simulink model "Wanderwellen_Leitungsmodell"  (R2022a)
settings: Solver=VariableStepAuto  StartTime=0.0  StopTime=0.05  RelTol=1e-3
model workspace (MAT data in the model file):
  C_impedanz = 1
  C_quelle = 1
  Delta_C = 2e-09
  Delta_G = 5000000
  Delta_L = 0.000228
  Delta_R = 0.048
  L_impedanz = 1
  L_quelle = 1
  R_impedanz = 0
  R_quelle = 0
  U = 20000
  U_type = 1
  Z_abschluss_type = 1
  Z_quelle_type = 1
  f = 50
  laenge = 0.2
  n_seg = 1
libraries: fl_lib x617, nesl_utility x207, ee_lib x3
(part 1 of 6)
settings Model: SimulationMode=rapid-accelerator  Creator=Arny  LastModifiedBy=stefa
settings SolverCC: AlgebraicLoopSolver=TrustRegion
settings DebuggingCC: UnconnectedInputMsg=warning  UnconnectedOutputMsg=warning  UnconnectedLineMsg=warning  SFMachineParentedDataDiag=warning
settings RTWCC: DLArmComputeVersion=19.05
settings SimscapeCC: SimscapeLogType=all  SimscapeLogSimulationStatistics=on  SimscapeLogName=simlog_leitungsmodell_3  SimscapeLogLimitData=off

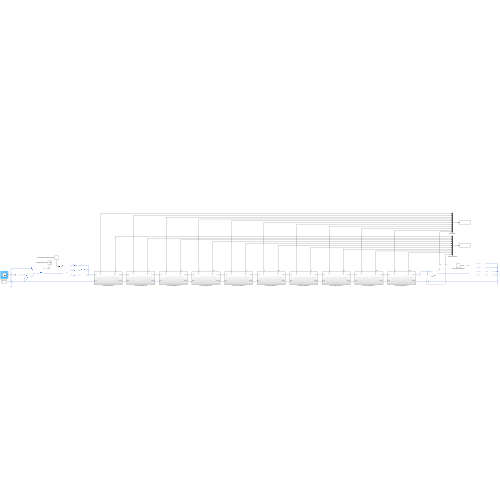
[thumbnail: Simulink's stored preview of the top-level diagram]
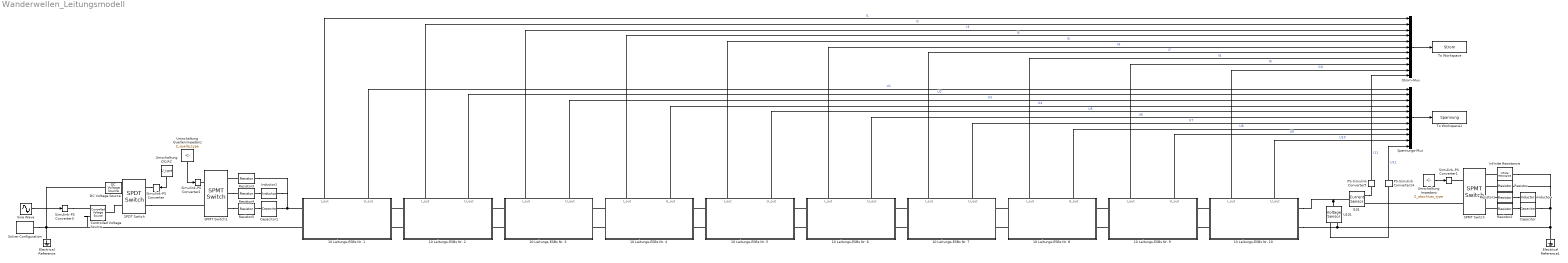
== system Wanderwellen_Leitungsmodell ==
  10 Leitungs-ESBs Nr. 1 : Subsystem
      settings: PortSchema="{\"entries\":[{\"content\":{\"sides\":[{\"content\":{\"connectorIds\":[\"LConn1\",\"LConn2\"]},\"type\":\"ConnectorPlacement.EquallySpacedRectSide\",\"uuid\":\"65052ebb-92dd-4621-bc28-5ee7f4d3a003\"},{\"content\":{\"connectorIds\":[\"RConn1\",\"RConn2\"],\"side\":\"RIGHT\"},\"type\":\"ConnectorPlacement.EquallySpacedRectSide\",\"uuid\":\"ad6a7191-e78a-426e-a776-ae1259ce905d\"},{\"content\":{\"connectorIds\":[\"Out1\",\"Out2\"],\"side\":\"TOP\"},\"type\":\"ConnectorPlacement.EquallySpacedRectSide\",\"uuid\":\"02566ec9-e537-49ed-9e06-af4a9095a538\"},{\"content\":{\"connectorIds\":[],\"side\":\"BOTTOM\"},\"type\":\"ConnectorPlacement.EquallySpacedRectSide\",\"uuid\":\"9e9501ed-61c6-491f-aa82-5958bb0ce8dc\"},{\"content\":{\"connectorIds\":[],\"side\":\"HIDDEN\"},\"type\":\"ConnectorPlacement.EquallySpacedRectSide\",\"uuid\":\"85703fc7-f421-416c-9ecd-4315fb8ade2d\"}]},\"type\":\"ConnectorPlacement.EquallySpacedConnector\",\"uuid\":\"39c1ec01-b535-48db-9665-193997bf92c2\"}],\"packageUris\":[\"http://schema.mathworks.com/mf0/Connector/R2020b\"],\"version\":\"1.0\"}"
  10 Leitungs-ESBs Nr. 10 : Subsystem
      settings: PortSchema="{\"entries\":[{\"content\":{\"sides\":[{\"content\":{\"connectorIds\":[\"LConn1\",\"LConn2\"]},\"type\":\"ConnectorPlacement.EquallySpacedRectSide\",\"uuid\":\"65052ebb-92dd-4621-bc28-5ee7f4d3a003\"},{\"content\":{\"connectorIds\":[\"RConn1\",\"RConn2\"],\"side\":\"RIGHT\"},\"type\":\"ConnectorPlacement.EquallySpacedRectSide\",\"uuid\":\"ad6a7191-e78a-426e-a776-ae1259ce905d\"},{\"content\":{\"connectorIds\":[\"Out1\",\"Out2\"],\"side\":\"TOP\"},\"type\":\"ConnectorPlacement.EquallySpacedRectSide\",\"uuid\":\"02566ec9-e537-49ed-9e06-af4a9095a538\"},{\"content\":{\"connectorIds\":[],\"side\":\"BOTTOM\"},\"type\":\"ConnectorPlacement.EquallySpacedRectSide\",\"uuid\":\"9e9501ed-61c6-491f-aa82-5958bb0ce8dc\"},{\"content\":{\"connectorIds\":[],\"side\":\"HIDDEN\"},\"type\":\"ConnectorPlacement.EquallySpacedRectSide\",\"uuid\":\"85703fc7-f421-416c-9ecd-4315fb8ade2d\"}]},\"type\":\"ConnectorPlacement.EquallySpacedConnector\",\"uuid\":\"39c1ec01-b535-48db-9665-193997bf92c2\"}],\"packageUris\":[\"http://schema.mathworks.com/mf0/Connector/R2020b\"],\"version\":\"1.0\"}"
  10 Leitungs-ESBs Nr. 2 : Subsystem
      settings: PortSchema="{\"entries\":[{\"content\":{\"sides\":[{\"content\":{\"connectorIds\":[\"LConn1\",\"LConn2\"]},\"type\":\"ConnectorPlacement.EquallySpacedRectSide\",\"uuid\":\"65052ebb-92dd-4621-bc28-5ee7f4d3a003\"},{\"content\":{\"connectorIds\":[\"RConn1\",\"RConn2\"],\"side\":\"RIGHT\"},\"type\":\"ConnectorPlacement.EquallySpacedRectSide\",\"uuid\":\"ad6a7191-e78a-426e-a776-ae1259ce905d\"},{\"content\":{\"connectorIds\":[\"Out1\",\"Out2\"],\"side\":\"TOP\"},\"type\":\"ConnectorPlacement.EquallySpacedRectSide\",\"uuid\":\"02566ec9-e537-49ed-9e06-af4a9095a538\"},{\"content\":{\"connectorIds\":[],\"side\":\"BOTTOM\"},\"type\":\"ConnectorPlacement.EquallySpacedRectSide\",\"uuid\":\"9e9501ed-61c6-491f-aa82-5958bb0ce8dc\"},{\"content\":{\"connectorIds\":[],\"side\":\"HIDDEN\"},\"type\":\"ConnectorPlacement.EquallySpacedRectSide\",\"uuid\":\"85703fc7-f421-416c-9ecd-4315fb8ade2d\"}]},\"type\":\"ConnectorPlacement.EquallySpacedConnector\",\"uuid\":\"39c1ec01-b535-48db-9665-193997bf92c2\"}],\"packageUris\":[\"http://schema.mathworks.com/mf0/Connector/R2020b\"],\"version\":\"1.0\"}"
  10 Leitungs-ESBs Nr. 3 : Subsystem
      settings: PortSchema="{\"entries\":[{\"content\":{\"sides\":[{\"content\":{\"connectorIds\":[\"LConn1\",\"LConn2\"]},\"type\":\"ConnectorPlacement.EquallySpacedRectSide\",\"uuid\":\"65052ebb-92dd-4621-bc28-5ee7f4d3a003\"},{\"content\":{\"connectorIds\":[\"RConn1\",\"RConn2\"],\"side\":\"RIGHT\"},\"type\":\"ConnectorPlacement.EquallySpacedRectSide\",\"uuid\":\"ad6a7191-e78a-426e-a776-ae1259ce905d\"},{\"content\":{\"connectorIds\":[\"Out1\",\"Out2\"],\"side\":\"TOP\"},\"type\":\"ConnectorPlacement.EquallySpacedRectSide\",\"uuid\":\"02566ec9-e537-49ed-9e06-af4a9095a538\"},{\"content\":{\"connectorIds\":[],\"side\":\"BOTTOM\"},\"type\":\"ConnectorPlacement.EquallySpacedRectSide\",\"uuid\":\"9e9501ed-61c6-491f-aa82-5958bb0ce8dc\"},{\"content\":{\"connectorIds\":[],\"side\":\"HIDDEN\"},\"type\":\"ConnectorPlacement.EquallySpacedRectSide\",\"uuid\":\"85703fc7-f421-416c-9ecd-4315fb8ade2d\"}]},\"type\":\"ConnectorPlacement.EquallySpacedConnector\",\"uuid\":\"39c1ec01-b535-48db-9665-193997bf92c2\"}],\"packageUris\":[\"http://schema.mathworks.com/mf0/Connector/R2020b\"],\"version\":\"1.0\"}"
  10 Leitungs-ESBs Nr. 4 : Subsystem
      settings: PortSchema="{\"entries\":[{\"content\":{\"sides\":[{\"content\":{\"connectorIds\":[\"LConn1\",\"LConn2\"]},\"type\":\"ConnectorPlacement.EquallySpacedRectSide\",\"uuid\":\"65052ebb-92dd-4621-bc28-5ee7f4d3a003\"},{\"content\":{\"connectorIds\":[\"RConn1\",\"RConn2\"],\"side\":\"RIGHT\"},\"type\":\"ConnectorPlacement.EquallySpacedRectSide\",\"uuid\":\"ad6a7191-e78a-426e-a776-ae1259ce905d\"},{\"content\":{\"connectorIds\":[\"Out1\",\"Out2\"],\"side\":\"TOP\"},\"type\":\"ConnectorPlacement.EquallySpacedRectSide\",\"uuid\":\"02566ec9-e537-49ed-9e06-af4a9095a538\"},{\"content\":{\"connectorIds\":[],\"side\":\"BOTTOM\"},\"type\":\"ConnectorPlacement.EquallySpacedRectSide\",\"uuid\":\"9e9501ed-61c6-491f-aa82-5958bb0ce8dc\"},{\"content\":{\"connectorIds\":[],\"side\":\"HIDDEN\"},\"type\":\"ConnectorPlacement.EquallySpacedRectSide\",\"uuid\":\"85703fc7-f421-416c-9ecd-4315fb8ade2d\"}]},\"type\":\"ConnectorPlacement.EquallySpacedConnector\",\"uuid\":\"39c1ec01-b535-48db-9665-193997bf92c2\"}],\"packageUris\":[\"http://schema.mathworks.com/mf0/Connector/R2020b\"],\"version\":\"1.0\"}"
  10 Leitungs-ESBs Nr. 5 : Subsystem
      settings: PortSchema="{\"entries\":[{\"content\":{\"sides\":[{\"content\":{\"connectorIds\":[\"LConn1\",\"LConn2\"]},\"type\":\"ConnectorPlacement.EquallySpacedRectSide\",\"uuid\":\"65052ebb-92dd-4621-bc28-5ee7f4d3a003\"},{\"content\":{\"connectorIds\":[\"RConn1\",\"RConn2\"],\"side\":\"RIGHT\"},\"type\":\"ConnectorPlacement.EquallySpacedRectSide\",\"uuid\":\"ad6a7191-e78a-426e-a776-ae1259ce905d\"},{\"content\":{\"connectorIds\":[\"Out1\",\"Out2\"],\"side\":\"TOP\"},\"type\":\"ConnectorPlacement.EquallySpacedRectSide\",\"uuid\":\"02566ec9-e537-49ed-9e06-af4a9095a538\"},{\"content\":{\"connectorIds\":[],\"side\":\"BOTTOM\"},\"type\":\"ConnectorPlacement.EquallySpacedRectSide\",\"uuid\":\"9e9501ed-61c6-491f-aa82-5958bb0ce8dc\"},{\"content\":{\"connectorIds\":[],\"side\":\"HIDDEN\"},\"type\":\"ConnectorPlacement.EquallySpacedRectSide\",\"uuid\":\"85703fc7-f421-416c-9ecd-4315fb8ade2d\"}]},\"type\":\"ConnectorPlacement.EquallySpacedConnector\",\"uuid\":\"39c1ec01-b535-48db-9665-193997bf92c2\"}],\"packageUris\":[\"http://schema.mathworks.com/mf0/Connector/R2020b\"],\"version\":\"1.0\"}"
  10 Leitungs-ESBs Nr. 6 : Subsystem
      settings: PortSchema="{\"entries\":[{\"content\":{\"sides\":[{\"content\":{\"connectorIds\":[\"LConn1\",\"LConn2\"]},\"type\":\"ConnectorPlacement.EquallySpacedRectSide\",\"uuid\":\"65052ebb-92dd-4621-bc28-5ee7f4d3a003\"},{\"content\":{\"connectorIds\":[\"RConn1\",\"RConn2\"],\"side\":\"RIGHT\"},\"type\":\"ConnectorPlacement.EquallySpacedRectSide\",\"uuid\":\"ad6a7191-e78a-426e-a776-ae1259ce905d\"},{\"content\":{\"connectorIds\":[\"Out1\",\"Out2\"],\"side\":\"TOP\"},\"type\":\"ConnectorPlacement.EquallySpacedRectSide\",\"uuid\":\"02566ec9-e537-49ed-9e06-af4a9095a538\"},{\"content\":{\"connectorIds\":[],\"side\":\"BOTTOM\"},\"type\":\"ConnectorPlacement.EquallySpacedRectSide\",\"uuid\":\"9e9501ed-61c6-491f-aa82-5958bb0ce8dc\"},{\"content\":{\"connectorIds\":[],\"side\":\"HIDDEN\"},\"type\":\"ConnectorPlacement.EquallySpacedRectSide\",\"uuid\":\"85703fc7-f421-416c-9ecd-4315fb8ade2d\"}]},\"type\":\"ConnectorPlacement.EquallySpacedConnector\",\"uuid\":\"39c1ec01-b535-48db-9665-193997bf92c2\"}],\"packageUris\":[\"http://schema.mathworks.com/mf0/Connector/R2020b\"],\"version\":\"1.0\"}"
  10 Leitungs-ESBs Nr. 7 : Subsystem
      settings: PortSchema="{\"entries\":[{\"content\":{\"sides\":[{\"content\":{\"connectorIds\":[\"LConn1\",\"LConn2\"]},\"type\":\"ConnectorPlacement.EquallySpacedRectSide\",\"uuid\":\"65052ebb-92dd-4621-bc28-5ee7f4d3a003\"},{\"content\":{\"connectorIds\":[\"RConn1\",\"RConn2\"],\"side\":\"RIGHT\"},\"type\":\"ConnectorPlacement.EquallySpacedRectSide\",\"uuid\":\"ad6a7191-e78a-426e-a776-ae1259ce905d\"},{\"content\":{\"connectorIds\":[\"Out1\",\"Out2\"],\"side\":\"TOP\"},\"type\":\"ConnectorPlacement.EquallySpacedRectSide\",\"uuid\":\"02566ec9-e537-49ed-9e06-af4a9095a538\"},{\"content\":{\"connectorIds\":[],\"side\":\"BOTTOM\"},\"type\":\"ConnectorPlacement.EquallySpacedRectSide\",\"uuid\":\"9e9501ed-61c6-491f-aa82-5958bb0ce8dc\"},{\"content\":{\"connectorIds\":[],\"side\":\"HIDDEN\"},\"type\":\"ConnectorPlacement.EquallySpacedRectSide\",\"uuid\":\"85703fc7-f421-416c-9ecd-4315fb8ade2d\"}]},\"type\":\"ConnectorPlacement.EquallySpacedConnector\",\"uuid\":\"39c1ec01-b535-48db-9665-193997bf92c2\"}],\"packageUris\":[\"http://schema.mathworks.com/mf0/Connector/R2020b\"],\"version\":\"1.0\"}"
  10 Leitungs-ESBs Nr. 8 : Subsystem
      settings: PortSchema="{\"entries\":[{\"content\":{\"sides\":[{\"content\":{\"connectorIds\":[\"LConn1\",\"LConn2\"]},\"type\":\"ConnectorPlacement.EquallySpacedRectSide\",\"uuid\":\"65052ebb-92dd-4621-bc28-5ee7f4d3a003\"},{\"content\":{\"connectorIds\":[\"RConn1\",\"RConn2\"],\"side\":\"RIGHT\"},\"type\":\"ConnectorPlacement.EquallySpacedRectSide\",\"uuid\":\"ad6a7191-e78a-426e-a776-ae1259ce905d\"},{\"content\":{\"connectorIds\":[\"Out1\",\"Out2\"],\"side\":\"TOP\"},\"type\":\"ConnectorPlacement.EquallySpacedRectSide\",\"uuid\":\"02566ec9-e537-49ed-9e06-af4a9095a538\"},{\"content\":{\"connectorIds\":[],\"side\":\"BOTTOM\"},\"type\":\"ConnectorPlacement.EquallySpacedRectSide\",\"uuid\":\"9e9501ed-61c6-491f-aa82-5958bb0ce8dc\"},{\"content\":{\"connectorIds\":[],\"side\":\"HIDDEN\"},\"type\":\"ConnectorPlacement.EquallySpacedRectSide\",\"uuid\":\"85703fc7-f421-416c-9ecd-4315fb8ade2d\"}]},\"type\":\"ConnectorPlacement.EquallySpacedConnector\",\"uuid\":\"39c1ec01-b535-48db-9665-193997bf92c2\"}],\"packageUris\":[\"http://schema.mathworks.com/mf0/Connector/R2020b\"],\"version\":\"1.0\"}"
  10 Leitungs-ESBs Nr. 9 : Subsystem
      settings: PortSchema="{\"entries\":[{\"content\":{\"sides\":[{\"content\":{\"connectorIds\":[\"LConn1\",\"LConn2\"]},\"type\":\"ConnectorPlacement.EquallySpacedRectSide\",\"uuid\":\"65052ebb-92dd-4621-bc28-5ee7f4d3a003\"},{\"content\":{\"connectorIds\":[\"RConn1\",\"RConn2\"],\"side\":\"RIGHT\"},\"type\":\"ConnectorPlacement.EquallySpacedRectSide\",\"uuid\":\"ad6a7191-e78a-426e-a776-ae1259ce905d\"},{\"content\":{\"connectorIds\":[\"Out1\",\"Out2\"],\"side\":\"TOP\"},\"type\":\"ConnectorPlacement.EquallySpacedRectSide\",\"uuid\":\"02566ec9-e537-49ed-9e06-af4a9095a538\"},{\"content\":{\"connectorIds\":[],\"side\":\"BOTTOM\"},\"type\":\"ConnectorPlacement.EquallySpacedRectSide\",\"uuid\":\"9e9501ed-61c6-491f-aa82-5958bb0ce8dc\"},{\"content\":{\"connectorIds\":[],\"side\":\"HIDDEN\"},\"type\":\"ConnectorPlacement.EquallySpacedRectSide\",\"uuid\":\"85703fc7-f421-416c-9ecd-4315fb8ade2d\"}]},\"type\":\"ConnectorPlacement.EquallySpacedConnector\",\"uuid\":\"39c1ec01-b535-48db-9665-193997bf92c2\"}],\"packageUris\":[\"http://schema.mathworks.com/mf0/Connector/R2020b\"],\"version\":\"1.0\"}"
  Capacitor : fl_lib/Electrical/Electrical Elements/Capacitor  c=C_impedanz F  r=0 Ohm  g=0 1/Ohm  i_specify=off  i_priority=None  i=0 A  i_nominal_specify=off  i_nominal_unit=A  i_nominal_value=1  v_specify=off  v_priority=None  v=0 V  v_nominal_specify=off  v_nominal_unit=V  v_nominal_value=1  vc_specify=off  vc_priority=High  vc=0 V  vc_nominal_specify=off  vc_nominal_unit=V  vc_nominal_value=1
      settings: SourceProductBaseCode=PW,SS,VE
  Capacitor1 : fl_lib/Electrical/Electrical Elements/Capacitor  c=C_quelle F  r=0 Ohm  g=0 1/Ohm  i_specify=off  i_priority=None  i=0 A  i_nominal_specify=off  i_nominal_unit=A  i_nominal_value=1  v_specify=off  v_priority=None  v=0 V  v_nominal_specify=off  v_nominal_unit=V  v_nominal_value=1  vc_specify=off  vc_priority=High  vc=0 V  vc_nominal_specify=off  vc_nominal_unit=V  vc_nominal_value=1
      settings: SourceProductBaseCode=PW,SS,VE
  Controlled Voltage Source : fl_lib/Electrical/Electrical Sources/Controlled Voltage Source
      settings: SourceProductBaseCode=PW,SS,VE
  DC Voltage Source : fl_lib/Electrical/Electrical Sources/DC Voltage Source  v0=U V
      settings: SourceProductBaseCode=PW,SS,VE
  Electrical Reference : fl_lib/Electrical/Electrical Elements/Electrical Reference
      settings: SourceProductBaseCode=PW,SS,VE
  Electrical Reference1 : fl_lib/Electrical/Electrical Elements/Electrical Reference
      settings: SourceProductBaseCode=PW,SS,VE
  I101 : fl_lib/Electrical/Electrical Sensors/Current Sensor
      settings: SourceProductBaseCode=PW,SS,VE
  Inductor : fl_lib/Electrical/Electrical Elements/Inductor  l=L_impedanz H  r=0 Ohm  g=0 1/Ohm  i_specify=off  i_priority=None  i=0 A  i_nominal_specify=off  i_nominal_unit=A  i_nominal_value=1  v_specify=off  v_priority=None  v=0 V  v_nominal_specify=off  v_nominal_unit=V  v_nominal_value=1  i_L_specify=off  i_L_priority=High  i_L=0 A  i_L_nominal_specify=off  i_L_nominal_unit=A  i_L_nominal_value=1
      settings: SourceProductBaseCode=PW,SS,VE
  Inductor1 : fl_lib/Electrical/Electrical Elements/Inductor  l=L_quelle H  r=0 Ohm  g=0 1/Ohm  i_specify=off  i_priority=None  i=0 A  i_nominal_specify=off  i_nominal_unit=A  i_nominal_value=1  v_specify=off  v_priority=None  v=0 V  v_nominal_specify=off  v_nominal_unit=V  v_nominal_value=1  i_L_specify=off  i_L_priority=High  i_L=0 A  i_L_nominal_specify=off  i_L_nominal_unit=A  i_L_nominal_value=1
      settings: SourceProductBaseCode=PW,SS,VE
  Infinite Resistance : fl_lib/Electrical/Electrical Elements/Infinite Resistance  v_specify=off  v_priority=None  v=0 V  v_nominal_specify=off  v_nominal_unit=V  v_nominal_value=1
      settings: SourceProductBaseCode=PW,SS,VE  InternalSimscapePortConfiguration="{\"Bottom\":[],\"Left\":[{\"id\":\"p\",\"label\":\"+\",\"type\":\"foundation.electrical.electrical\"}],\"Right\":[{\"id\":\"n\",\"label\":\"-\",\"type\":\"foundation.electrical.electrical\"}],\"Top\":[]}"
  PS-Simulink Converter14 : nesl_utility/PS-Simulink Converter  PhysicalDomain=network_engine_domain  SubClassName=ps_output  LeftPortType=input  RightPortType=output  PseudoPeriodic=off  Frequencies=[]  VectorFormat=1-D array  Unit=inherit  AffineConversion=off
      settings: SourceProductBaseCode=SS,PW,VE
  PS-Simulink Converter5 : nesl_utility/PS-Simulink Converter  PhysicalDomain=network_engine_domain  SubClassName=ps_output  LeftPortType=input  RightPortType=output  PseudoPeriodic=off  Frequencies=[]  VectorFormat=1-D array  Unit=inherit  AffineConversion=off
      settings: SourceProductBaseCode=SS,PW,VE
  Resistor : fl_lib/Electrical/Electrical Elements/Resistor  R=R_impedanz Ohm  i_specify=off  i_priority=None  i=0 A  i_nominal_specify=off  i_nominal_unit=A  i_nominal_value=1  v_specify=off  v_priority=None  v=0 V  v_nominal_specify=off  v_nominal_unit=V  v_nominal_value=1
      settings: SourceProductBaseCode=PW,SS,VE
  Resistor1 : fl_lib/Electrical/Electrical Elements/Resistor  R=R_impedanz Ohm  i_specify=off  i_priority=None  i=0 A  i_nominal_specify=off  i_nominal_unit=A  i_nominal_value=1  v_specify=off  v_priority=None  v=0 V  v_nominal_specify=off  v_nominal_unit=V  v_nominal_value=1
      settings: SourceProductBaseCode=PW,SS,VE
  Resistor2 : fl_lib/Electrical/Electrical Elements/Resistor  R=R_impedanz Ohm  i_specify=off  i_priority=None  i=0 A  i_nominal_specify=off  i_nominal_unit=A  i_nominal_value=1  v_specify=off  v_priority=None  v=0 V  v_nominal_specify=off  v_nominal_unit=V  v_nominal_value=1
      settings: SourceProductBaseCode=PW,SS,VE
  Resistor3 : fl_lib/Electrical/Electrical Elements/Resistor  R=R_quelle Ohm  i_specify=off  i_priority=None  i=0 A  i_nominal_specify=off  i_nominal_unit=A  i_nominal_value=1  v_specify=off  v_priority=None  v=0 V  v_nominal_specify=off  v_nominal_unit=V  v_nominal_value=1
      settings: SourceProductBaseCode=PW,SS,VE
  Resistor4 : fl_lib/Electrical/Electrical Elements/Resistor  R=R_quelle Ohm  i_specify=off  i_priority=None  i=0 A  i_nominal_specify=off  i_nominal_unit=A  i_nominal_value=1  v_specify=off  v_priority=None  v=0 V  v_nominal_specify=off  v_nominal_unit=V  v_nominal_value=1
      settings: SourceProductBaseCode=PW,SS,VE
  Resistor5 : fl_lib/Electrical/Electrical Elements/Resistor  R=R_quelle Ohm  i_specify=off  i_priority=None  i=0 A  i_nominal_specify=off  i_nominal_unit=A  i_nominal_value=1  v_specify=off  v_priority=None  v=0 V  v_nominal_specify=off  v_nominal_unit=V  v_nominal_value=1
      settings: SourceProductBaseCode=PW,SS,VE
  SPDT Switch : ee_lib/Switches & Breakers/SPDT Switch  R_closed=0.01 Ohm  G_open=1e-6 S  Threshold=0.5 V  Width=0 V  model_dynamics=0  t_on=1e-3 s  t_off=1e-3 s  initial_vT=0 V
      settings: SourceProductBaseCode=PS
  SPMT Switch : ee_lib/Switches & Breakers/SPMT Switch  number_throws=ee.enum.switches.numberThrows.four  R_closed=0.01 Ohm  G_open=1e-6 S  enable_fault=simscape.enum.onoff.off  fault_action=simscape.enum.assert.action.none  fault_trigger=ee.enum.faults.faultTrigger.temporal  t_fault=1 s  max_permissible_current=inf A  t_fail_on_current=1 s
      settings: SourceProductBaseCode=PS  InternalSimscapePortConfiguration="{\"Bottom\":[],\"Left\":[{\"id\":\"vT\",\"label\":\"vT\",\"type\":\"input\"},{\"id\":\"p\",\"label\":\"\",\"type\":\"foundation.electrical.electrical\"}],\"Right\":[{\"id\":\"n1\",\"label\":\"\",\"type\":\"foundation.electrical.electrical\"},{\"id\":\"n2\",\"label\":\"\",\"type\":\"foundation.electrical.electrical\"},{\"id\":\"n3\",\"label\":\"\",\"type\":\"foundation.electrical.electrical\"},{\"id\":\"n4\",\"label\":\"\",\"type\":\"foundation.electrical.electrical\"}],\"Top\":[]}"
  SPMT Switch1 : ee_lib/Switches & Breakers/SPMT Switch  number_throws=ee.enum.switches.numberThrows.three  R_closed=0.01 Ohm  G_open=1e-6 S  enable_fault=simscape.enum.onoff.off  fault_action=simscape.enum.assert.action.none  fault_trigger=ee.enum.faults.faultTrigger.temporal  t_fault=1 s  max_permissible_current=inf A  t_fail_on_current=1 s
      settings: SourceProductBaseCode=PS  InternalSimscapePortConfiguration="{\"Bottom\":[],\"Left\":[{\"id\":\"vT\",\"label\":\"vT\",\"type\":\"input\"},{\"id\":\"p\",\"label\":\"\",\"type\":\"foundation.electrical.electrical\"}],\"Right\":[{\"id\":\"n1\",\"label\":\"\",\"type\":\"foundation.electrical.electrical\"},{\"id\":\"n2\",\"label\":\"\",\"type\":\"foundation.electrical.electrical\"},{\"id\":\"n3\",\"label\":\"\",\"type\":\"foundation.electrical.electrical\"}],\"Top\":[]}"
  Simulink-PS Converter{,1..3} (4 alike) : nesl_utility/Simulink-PS Converter  PhysicalDomain=network_engine_domain  SubClassName=ps_input  LeftPortType=input  RightPortType=output  PseudoPeriodic=off  Frequencies=[]  NoiseDistribution=none  NoiseParameters=[]  Unit=1  AffineConversion=off  FilteringAndDerivatives=provide  SimscapeFilterOrder=1  InputFilterTimeConstant=0.001  UdotUserProvided=0
      settings: SourceProductBaseCode=SS,PW,VE
  Sine Wave : Sin  Amplitude=sqrt(2)*U  Frequency=2*pi*f  SampleTime=0
  Solver Configuration : nesl_utility/Solver Configuration  PhysicalDomain=network_engine_domain  SubClassName=solver  LeftPortType=input  RightPortType=generic  Tones=[]  Harmonics=[]  SimulateNoise=off  Profile=off  UseLocalSampling=off  EnableSwitchedLinearOptims=on  FrequencyDomain=off  UseCCode=off  RelTol=0.001  AbsTol=1e-06  MinStep=1e-09  ToWorkspace=off  RevertToSquareIcSolve=off  NumHomotopyIterations=100  PhasorMode=off  PhasorModeNumHarmonics=1  IndexReductionMethod=DerivativeReplacement  DoDC=off  ResidualTolerance=1e-09  UseLocalSolver=off  LocalSolverChoice=NE_BACKWARD_EULER_ADVANCER  LocalSolverSampleTime=0.001  DoFixedCost=off  MaxNonlinIter=3  MaxModeIter=2  ComputeImpulses=off  ImpulseIterations=2  LinearAlgebra=auto  LinearAlgebraNumThread=0  EquationFormulation=NE_TIME_EF  DelaysMemoryBudget=1024  AutomaticFiltering=on  FilteringTimeConstant=0.001  PartitionStorageMethod=AS_NEEDED  PartitionMemoryBudget=1024  PartitionMethod=ROBUST
      settings: SourceProductBaseCode=SS,PW,VE
  Spannungs-Mux : Mux  Inputs=11
  Strom-Mux : Mux  Inputs=11
  To Workspace : ToWorkspace  VariableName=Strom  SaveFormat=Structure  SampleTime=-1
  To Workspace1 : ToWorkspace  VariableName=Spannung  SaveFormat=Structure  SampleTime=-1
  U101 : fl_lib/Electrical/Electrical Sensors/Voltage Sensor
      settings: SourceProductBaseCode=PW,SS,VE
  Umschaltung DC/AC : Constant  Value=U_type  VectorParams1D=off
  Umschaltung Impedanz : Constant  Value=Z_abschluss_type  VectorParams1D=off
  Umschaltung Quellenimpedanz : Constant  Value=Z_quelle_type  VectorParams1D=off
  wires:
  10 Leitungs-ESBs Nr. 1/1(I_out) -> Strom-Mux/1  "I1"
  10 Leitungs-ESBs Nr. 2/1(I_out) -> Strom-Mux/2  "I2"
  10 Leitungs-ESBs Nr. 3/1(I_out) -> Strom-Mux/3  "I3"
  10 Leitungs-ESBs Nr. 4/1(I_out) -> Strom-Mux/4  "I4"
  10 Leitungs-ESBs Nr. 5/1(I_out) -> Strom-Mux/5  "I5"
  10 Leitungs-ESBs Nr. 6/1(I_out) -> Strom-Mux/6  "I6"
  10 Leitungs-ESBs Nr. 7/1(I_out) -> Strom-Mux/7  "I7"
  10 Leitungs-ESBs Nr. 8/1(I_out) -> Strom-Mux/8  "I8"
  10 Leitungs-ESBs Nr. 9/1(I_out) -> Strom-Mux/9  "I9"
  10 Leitungs-ESBs Nr. 10/1(I_out) -> Strom-Mux/10  "I10"
  PS-Simulink Converter5/1 -> Strom-Mux/11  "I11"
  10 Leitungs-ESBs Nr. 1/2(U_out) -> Spannungs-Mux/1  "U1"
  10 Leitungs-ESBs Nr. 2/2(U_out) -> Spannungs-Mux/2  "U2"
  10 Leitungs-ESBs Nr. 3/2(U_out) -> Spannungs-Mux/3  "U3"
  10 Leitungs-ESBs Nr. 4/2(U_out) -> Spannungs-Mux/4  "U4"
  10 Leitungs-ESBs Nr. 5/2(U_out) -> Spannungs-Mux/5  "U5"
  10 Leitungs-ESBs Nr. 6/2(U_out) -> Spannungs-Mux/6  "U6"
  10 Leitungs-ESBs Nr. 7/2(U_out) -> Spannungs-Mux/7  "U7"
  10 Leitungs-ESBs Nr. 8/2(U_out) -> Spannungs-Mux/8  "U8"
  10 Leitungs-ESBs Nr. 9/2(U_out) -> Spannungs-Mux/9  "U9"
  10 Leitungs-ESBs Nr. 10/2(U_out) -> Spannungs-Mux/10  "U10"
  PS-Simulink Converter14/1 -> Spannungs-Mux/11  "U11"
  Strom-Mux/1 -> To Workspace/1
  Spannungs-Mux/1 -> To Workspace1/1
  Umschaltung DC/AC/1 -> Simulink-PS Converter/1
  Umschaltung Impedanz/1 -> Simulink-PS Converter1/1
  Umschaltung Quellenimpedanz/1 -> Simulink-PS Converter2/1
  Sine Wave/1 -> Simulink-PS Converter3/1
  connections:
  Solver Configuration/RConn1 -- DC Voltage Source/RConn1 -- Controlled Voltage Source/RConn2 -- 10 Leitungs-ESBs Nr. 1/LConn2 -- Electrical Reference/LConn1
  10 Leitungs-ESBs Nr. 2/LConn1 -- 10 Leitungs-ESBs Nr. 1/RConn1
  10 Leitungs-ESBs Nr. 2/LConn2 -- 10 Leitungs-ESBs Nr. 1/RConn2
  10 Leitungs-ESBs Nr. 3/LConn1 -- 10 Leitungs-ESBs Nr. 2/RConn1
  10 Leitungs-ESBs Nr. 3/LConn2 -- 10 Leitungs-ESBs Nr. 2/RConn2
  10 Leitungs-ESBs Nr. 4/LConn2 -- 10 Leitungs-ESBs Nr. 3/RConn2
  10 Leitungs-ESBs Nr. 4/LConn1 -- 10 Leitungs-ESBs Nr. 3/RConn1
  10 Leitungs-ESBs Nr. 5/LConn2 -- 10 Leitungs-ESBs Nr. 4/RConn2
  10 Leitungs-ESBs Nr. 5/LConn1 -- 10 Leitungs-ESBs Nr. 4/RConn1
  10 Leitungs-ESBs Nr. 6/LConn2 -- 10 Leitungs-ESBs Nr. 5/RConn2
  10 Leitungs-ESBs Nr. 6/LConn1 -- 10 Leitungs-ESBs Nr. 5/RConn1
  10 Leitungs-ESBs Nr. 7/LConn2 -- 10 Leitungs-ESBs Nr. 6/RConn2
  10 Leitungs-ESBs Nr. 7/LConn1 -- 10 Leitungs-ESBs Nr. 6/RConn1
  10 Leitungs-ESBs Nr. 8/LConn2 -- 10 Leitungs-ESBs Nr. 7/RConn2
  10 Leitungs-ESBs Nr. 8/LConn1 -- 10 Leitungs-ESBs Nr. 7/RConn1
  10 Leitungs-ESBs Nr. 9/LConn2 -- 10 Leitungs-ESBs Nr. 8/RConn2
  10 Leitungs-ESBs Nr. 9/LConn1 -- 10 Leitungs-ESBs Nr. 8/RConn1
  10 Leitungs-ESBs Nr. 10/LConn2 -- 10 Leitungs-ESBs Nr. 9/RConn2
  10 Leitungs-ESBs Nr. 10/LConn1 -- 10 Leitungs-ESBs Nr. 9/RConn1
  U101/LConn1 -- 10 Leitungs-ESBs Nr. 10/RConn1 -- I101/LConn1
  U101/RConn2 -- 10 Leitungs-ESBs Nr. 10/RConn2 -- Inductor/RConn1 -- Resistor/RConn1 -- Infinite Resistance/RConn1 -- Capacitor/RConn1 -- Electrical Reference1/LConn1
  I101/RConn1 -- PS-Simulink Converter5/LConn1
  U101/RConn1 -- PS-Simulink Converter14/LConn1
  SPDT Switch/LConn1 -- Simulink-PS Converter/RConn1
  DC Voltage Source/LConn1 -- SPDT Switch/RConn1
  SPMT Switch/LConn2 -- I101/RConn2
  SPMT Switch/LConn1 -- Simulink-PS Converter1/RConn1
  Infinite Resistance/LConn1 -- SPMT Switch/RConn1
  Resistor/LConn1 -- SPMT Switch/RConn2
  Resistor1/LConn1 -- SPMT Switch/RConn3
  Resistor1/RConn1 -- Inductor/LConn1
  Resistor2/LConn1 -- SPMT Switch/RConn4
  Resistor2/RConn1 -- Capacitor/LConn1
  SPMT Switch1/LConn1 -- Simulink-PS Converter2/RConn1
  Resistor5/RConn1 -- Capacitor1/LConn1
  Resistor4/RConn1 -- Inductor1/LConn1
  SPMT Switch1/RConn3 -- Resistor5/LConn1
  Resistor3/LConn1 -- SPMT Switch1/RConn1
  SPMT Switch1/RConn2 -- Resistor4/LConn1
  Capacitor1/RConn1 -- Resistor3/RConn1 -- Inductor1/RConn1 -- 10 Leitungs-ESBs Nr. 1/LConn1
  SPDT Switch/LConn2 -- SPMT Switch1/LConn2
  Simulink-PS Converter3/RConn1 -- Controlled Voltage Source/RConn1
  SPDT Switch/RConn2 -- Controlled Voltage Source/LConn1

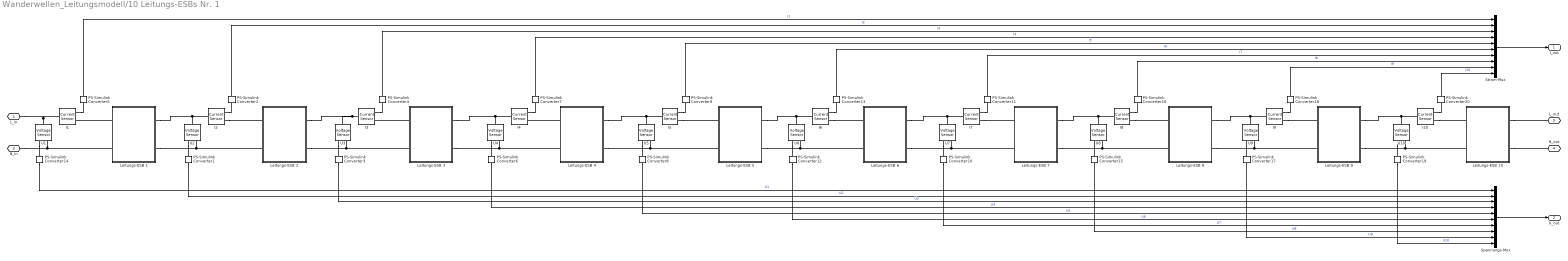
== system Wanderwellen_Leitungsmodell/10 Leitungs-ESBs Nr. 1 ==
  I{1..10} (10 alike) : fl_lib/Electrical/Electrical Sensors/Current Sensor
      settings: SourceProductBaseCode=PW,SS,VE
  Leitungs-ESB 1 : Subsystem
  Leitungs-ESB 10 : Subsystem
  Leitungs-ESB 2 : Subsystem
  Leitungs-ESB 3 : Subsystem
  Leitungs-ESB 4 : Subsystem
  Leitungs-ESB 5 : Subsystem
  Leitungs-ESB 6 : Subsystem
  Leitungs-ESB 7 : Subsystem
  Leitungs-ESB 8 : Subsystem
  Leitungs-ESB 9 : Subsystem
  PS-Simulink Converter{1..20} (20 alike) : nesl_utility/PS-Simulink Converter  PhysicalDomain=network_engine_domain  SubClassName=ps_output  LeftPortType=input  RightPortType=output  PseudoPeriodic=off  Frequencies=[]  VectorFormat=1-D array  Unit=inherit  AffineConversion=off
      settings: SourceProductBaseCode=SS,PW,VE
  Spannungs-Mux : Mux  Inputs=10
  Strom-Mux : Mux  Inputs=10
  U{1..10} (10 alike) : fl_lib/Electrical/Electrical Sensors/Voltage Sensor
      settings: SourceProductBaseCode=PW,SS,VE
  L_in : PMIOPort  Side=Left
  N_in : PMIOPort  Port=2  Side=Left
  L_out : PMIOPort  Port=3  Side=Right
  N_out : PMIOPort  Port=4  Side=Right
  I_out : Outport
  U_out : Outport  Port=2
  wires:
  PS-Simulink Converter5/1 -> Strom-Mux/1  "I1"
  PS-Simulink Converter2/1 -> Strom-Mux/2  "I2"
  PS-Simulink Converter4/1 -> Strom-Mux/3  "I3"
  PS-Simulink Converter7/1 -> Strom-Mux/4  "I4"
  PS-Simulink Converter9/1 -> Strom-Mux/5  "I5"
  PS-Simulink Converter13/1 -> Strom-Mux/6  "I6"
  PS-Simulink Converter11/1 -> Strom-Mux/7  "I7"
  PS-Simulink Converter16/1 -> Strom-Mux/8  "I8"
  PS-Simulink Converter18/1 -> Strom-Mux/9  "I9"
  PS-Simulink Converter20/1 -> Strom-Mux/10  "I10"
  PS-Simulink Converter19/1 -> Spannungs-Mux/10  "U10"
  PS-Simulink Converter17/1 -> Spannungs-Mux/9  "U9"
  PS-Simulink Converter15/1 -> Spannungs-Mux/8  "U8"
  PS-Simulink Converter10/1 -> Spannungs-Mux/7  "U7"
  PS-Simulink Converter12/1 -> Spannungs-Mux/6  "U6"
  PS-Simulink Converter8/1 -> Spannungs-Mux/5  "U5"
  PS-Simulink Converter6/1 -> Spannungs-Mux/4  "U4"
  PS-Simulink Converter3/1 -> Spannungs-Mux/3  "U3"
  PS-Simulink Converter1/1 -> Spannungs-Mux/2  "U2"
  PS-Simulink Converter14/1 -> Spannungs-Mux/1  "U1"
  Strom-Mux/1 -> I_out/1
  Spannungs-Mux/1 -> U_out/1
  connections:
  U1/LConn1 -- L_in/RConn1 -- I1/LConn1
  N_in/RConn1 -- U1/RConn2 -- Leitungs-ESB 1/LConn2
  Leitungs-ESB 1/LConn1 -- I1/RConn2
  I1/RConn1 -- PS-Simulink Converter5/LConn1
  U1/RConn1 -- PS-Simulink Converter14/LConn1
  Leitungs-ESB 2/LConn2 -- Leitungs-ESB 1/RConn2 -- U2/RConn2
  I2/LConn1 -- Leitungs-ESB 1/RConn1 -- U2/LConn1
  I2/RConn1 -- PS-Simulink Converter2/LConn1
  U2/RConn1 -- PS-Simulink Converter1/LConn1
  Leitungs-ESB 3/LConn2 -- Leitungs-ESB 2/RConn2 -- U3/RConn2
  I3/LConn1 -- Leitungs-ESB 2/RConn1 -- U3/LConn1
  I3/RConn1 -- PS-Simulink Converter4/LConn1
  U3/RConn1 -- PS-Simulink Converter3/LConn1
  Leitungs-ESB 3/LConn1 -- I3/RConn2
  Leitungs-ESB 3/RConn2 -- Leitungs-ESB 4/LConn2 -- U4/RConn2
  U4/LConn1 -- Leitungs-ESB 3/RConn1 -- I4/LConn1
  I4/RConn1 -- PS-Simulink Converter7/LConn1
  U4/RConn1 -- PS-Simulink Converter6/LConn1
  Leitungs-ESB 4/RConn2 -- U5/RConn2 -- Leitungs-ESB 5/LConn2
  Leitungs-ESB 4/RConn1 -- U5/LConn1 -- I5/LConn1
  I5/RConn1 -- PS-Simulink Converter9/LConn1
  U5/RConn1 -- PS-Simulink Converter8/LConn1
  Leitungs-ESB 6/RConn2 -- U7/RConn2 -- Leitungs-ESB 7/LConn2
  Leitungs-ESB 6/RConn1 -- U7/LConn1 -- I7/LConn1
  I7/RConn1 -- PS-Simulink Converter11/LConn1
  U7/RConn1 -- PS-Simulink Converter10/LConn1
  Leitungs-ESB 5/RConn2 -- U6/RConn2 -- Leitungs-ESB 6/LConn2
  Leitungs-ESB 5/RConn1 -- U6/LConn1 -- I6/LConn1
  U6/RConn1 -- PS-Simulink Converter12/LConn1
  I6/RConn1 -- PS-Simulink Converter13/LConn1
  I6/RConn2 -- Leitungs-ESB 6/LConn1
  Leitungs-ESB 7/RConn2 -- U8/RConn2 -- Leitungs-ESB 8/LConn2
  Leitungs-ESB 7/RConn1 -- U8/LConn1 -- I8/LConn1
  I8/RConn1 -- PS-Simulink Converter16/LConn1
  U8/RConn1 -- PS-Simulink Converter15/LConn1
  Leitungs-ESB 8/RConn2 -- U9/RConn2 -- Leitungs-ESB 9/LConn2
  Leitungs-ESB 8/RConn1 -- U9/LConn1 -- I9/LConn1
  I9/RConn1 -- PS-Simulink Converter18/LConn1
  U9/RConn1 -- PS-Simulink Converter17/LConn1
  Leitungs-ESB 9/RConn2 -- Leitungs-ESB 10/LConn2 -- U10/RConn2
  Leitungs-ESB 9/RConn1 -- U10/LConn1 -- I10/LConn1
  I10/RConn1 -- PS-Simulink Converter20/LConn1
  U10/RConn1 -- PS-Simulink Converter19/LConn1
  Leitungs-ESB 10/RConn1 -- L_out/RConn1
  Leitungs-ESB 10/RConn2 -- N_out/RConn1
  I2/RConn2 -- Leitungs-ESB 2/LConn1
  Leitungs-ESB 4/LConn1 -- I4/RConn2
  I5/RConn2 -- Leitungs-ESB 5/LConn1
  I7/RConn2 -- Leitungs-ESB 7/LConn1
  I8/RConn2 -- Leitungs-ESB 8/LConn1
  I9/RConn2 -- Leitungs-ESB 9/LConn1
  I10/RConn2 -- Leitungs-ESB 10/LConn1

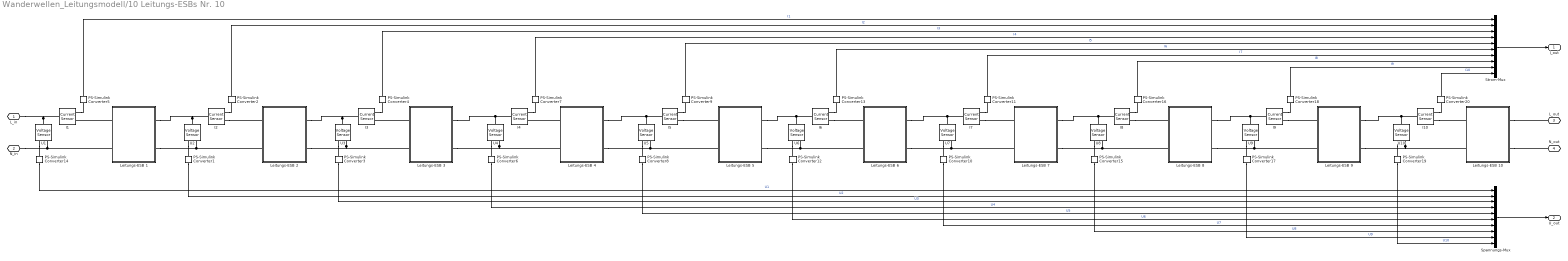
== system Wanderwellen_Leitungsmodell/10 Leitungs-ESBs Nr. 10 ==
  I{1..10} (10 alike) : fl_lib/Electrical/Electrical Sensors/Current Sensor
      settings: SourceProductBaseCode=PW,SS,VE
  Leitungs-ESB 1 : Subsystem
  Leitungs-ESB 10 : Subsystem
  Leitungs-ESB 2 : Subsystem
  Leitungs-ESB 3 : Subsystem
  Leitungs-ESB 4 : Subsystem
  Leitungs-ESB 5 : Subsystem
  Leitungs-ESB 6 : Subsystem
  Leitungs-ESB 7 : Subsystem
  Leitungs-ESB 8 : Subsystem
  Leitungs-ESB 9 : Subsystem
  PS-Simulink Converter{1..20} (20 alike) : nesl_utility/PS-Simulink Converter  PhysicalDomain=network_engine_domain  SubClassName=ps_output  LeftPortType=input  RightPortType=output  PseudoPeriodic=off  Frequencies=[]  VectorFormat=1-D array  Unit=inherit  AffineConversion=off
      settings: SourceProductBaseCode=SS,PW,VE
  Spannungs-Mux : Mux  Inputs=10
  Strom-Mux : Mux  Inputs=10
  U{1..10} (10 alike) : fl_lib/Electrical/Electrical Sensors/Voltage Sensor
      settings: SourceProductBaseCode=PW,SS,VE
  L_in : PMIOPort  Side=Left
  N_in : PMIOPort  Port=2  Side=Left
  L_out : PMIOPort  Port=3  Side=Right
  N_out : PMIOPort  Port=4  Side=Right
  I_out : Outport
  U_out : Outport  Port=2
  wires:
  PS-Simulink Converter5/1 -> Strom-Mux/1  "I1"
  PS-Simulink Converter2/1 -> Strom-Mux/2  "I2"
  PS-Simulink Converter4/1 -> Strom-Mux/3  "I3"
  PS-Simulink Converter7/1 -> Strom-Mux/4  "I4"
  PS-Simulink Converter9/1 -> Strom-Mux/5  "I5"
  PS-Simulink Converter13/1 -> Strom-Mux/6  "I6"
  PS-Simulink Converter11/1 -> Strom-Mux/7  "I7"
  PS-Simulink Converter16/1 -> Strom-Mux/8  "I8"
  PS-Simulink Converter18/1 -> Strom-Mux/9  "I9"
  PS-Simulink Converter20/1 -> Strom-Mux/10  "I10"
  PS-Simulink Converter19/1 -> Spannungs-Mux/10  "U10"
  PS-Simulink Converter17/1 -> Spannungs-Mux/9  "U9"
  PS-Simulink Converter15/1 -> Spannungs-Mux/8  "U8"
  PS-Simulink Converter10/1 -> Spannungs-Mux/7  "U7"
  PS-Simulink Converter12/1 -> Spannungs-Mux/6  "U6"
  PS-Simulink Converter8/1 -> Spannungs-Mux/5  "U5"
  PS-Simulink Converter6/1 -> Spannungs-Mux/4  "U4"
  PS-Simulink Converter3/1 -> Spannungs-Mux/3  "U3"
  PS-Simulink Converter1/1 -> Spannungs-Mux/2  "U2"
  PS-Simulink Converter14/1 -> Spannungs-Mux/1  "U1"
  Strom-Mux/1 -> I_out/1
  Spannungs-Mux/1 -> U_out/1
  connections:
  U1/LConn1 -- L_in/RConn1 -- I1/LConn1
  N_in/RConn1 -- Leitungs-ESB 1/LConn2 -- U1/RConn2
  Leitungs-ESB 1/LConn1 -- I1/RConn2
  I1/RConn1 -- PS-Simulink Converter5/LConn1
  U1/RConn1 -- PS-Simulink Converter14/LConn1
  Leitungs-ESB 2/LConn2 -- U2/RConn2 -- Leitungs-ESB 1/RConn2
  U2/LConn1 -- I2/LConn1 -- Leitungs-ESB 1/RConn1
  I2/RConn1 -- PS-Simulink Converter2/LConn1
  U2/RConn1 -- PS-Simulink Converter1/LConn1
  U3/RConn2 -- Leitungs-ESB 3/LConn2 -- Leitungs-ESB 2/RConn2
  U3/LConn1 -- I3/LConn1 -- Leitungs-ESB 2/RConn1
  I3/RConn1 -- PS-Simulink Converter4/LConn1
  U3/RConn1 -- PS-Simulink Converter3/LConn1
  Leitungs-ESB 3/LConn1 -- I3/RConn2
  U4/RConn2 -- Leitungs-ESB 3/RConn2 -- Leitungs-ESB 4/LConn2
  U4/LConn1 -- Leitungs-ESB 3/RConn1 -- I4/LConn1
  I4/RConn1 -- PS-Simulink Converter7/LConn1
  U4/RConn1 -- PS-Simulink Converter6/LConn1
  Leitungs-ESB 4/RConn2 -- Leitungs-ESB 5/LConn2 -- U5/RConn2
  Leitungs-ESB 4/RConn1 -- I5/LConn1 -- U5/LConn1
  I5/RConn1 -- PS-Simulink Converter9/LConn1
  U5/RConn1 -- PS-Simulink Converter8/LConn1
  Leitungs-ESB 6/RConn2 -- Leitungs-ESB 7/LConn2 -- U7/RConn2
  Leitungs-ESB 6/RConn1 -- I7/LConn1 -- U7/LConn1
  I7/RConn1 -- PS-Simulink Converter11/LConn1
  U7/RConn1 -- PS-Simulink Converter10/LConn1
  Leitungs-ESB 6/LConn2 -- Leitungs-ESB 5/RConn2 -- U6/RConn2
  Leitungs-ESB 5/RConn1 -- I6/LConn1 -- U6/LConn1
  U6/RConn1 -- PS-Simulink Converter12/LConn1
  I6/RConn1 -- PS-Simulink Converter13/LConn1
  I6/RConn2 -- Leitungs-ESB 6/LConn1
  Leitungs-ESB 8/LConn2 -- Leitungs-ESB 7/RConn2 -- U8/RConn2
  Leitungs-ESB 7/RConn1 -- I8/LConn1 -- U8/LConn1
  I8/RConn1 -- PS-Simulink Converter16/LConn1
  U8/RConn1 -- PS-Simulink Converter15/LConn1
  Leitungs-ESB 8/RConn2 -- Leitungs-ESB 9/LConn2 -- U9/RConn2
  Leitungs-ESB 8/RConn1 -- I9/LConn1 -- U9/LConn1
  I9/RConn1 -- PS-Simulink Converter18/LConn1
  U9/RConn1 -- PS-Simulink Converter17/LConn1
  U10/RConn2 -- Leitungs-ESB 9/RConn2 -- Leitungs-ESB 10/LConn2
  Leitungs-ESB 9/RConn1 -- I10/LConn1 -- U10/LConn1
  I10/RConn1 -- PS-Simulink Converter20/LConn1
  U10/RConn1 -- PS-Simulink Converter19/LConn1
  Leitungs-ESB 10/RConn1 -- L_out/RConn1
  Leitungs-ESB 10/RConn2 -- N_out/RConn1
  I2/RConn2 -- Leitungs-ESB 2/LConn1
  Leitungs-ESB 4/LConn1 -- I4/RConn2
  I5/RConn2 -- Leitungs-ESB 5/LConn1
  I7/RConn2 -- Leitungs-ESB 7/LConn1
  I8/RConn2 -- Leitungs-ESB 8/LConn1
  I9/RConn2 -- Leitungs-ESB 9/LConn1
  I10/RConn2 -- Leitungs-ESB 10/LConn1

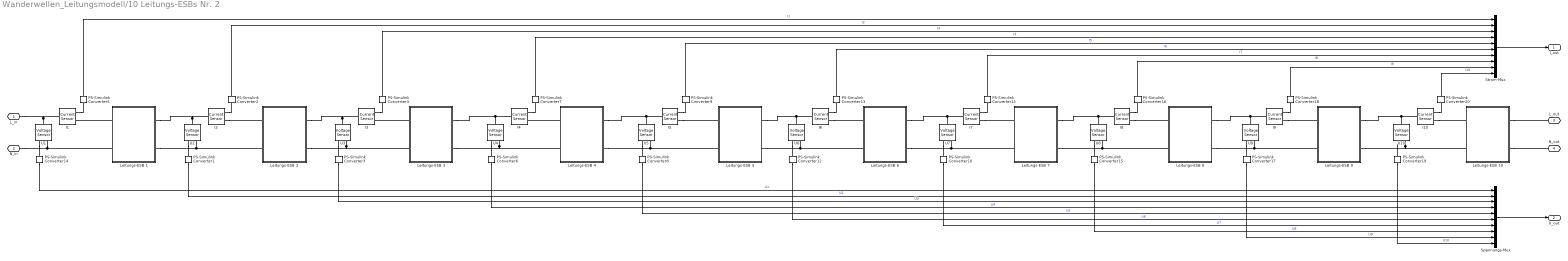
== system Wanderwellen_Leitungsmodell/10 Leitungs-ESBs Nr. 2 ==
  I{1..10} (10 alike) : fl_lib/Electrical/Electrical Sensors/Current Sensor
      settings: SourceProductBaseCode=PW,SS,VE
  Leitungs-ESB 1 : Subsystem
  Leitungs-ESB 10 : Subsystem
  Leitungs-ESB 2 : Subsystem
  Leitungs-ESB 3 : Subsystem
  Leitungs-ESB 4 : Subsystem
  Leitungs-ESB 5 : Subsystem
  Leitungs-ESB 6 : Subsystem
  Leitungs-ESB 7 : Subsystem
  Leitungs-ESB 8 : Subsystem
  Leitungs-ESB 9 : Subsystem
  PS-Simulink Converter{1..20} (20 alike) : nesl_utility/PS-Simulink Converter  PhysicalDomain=network_engine_domain  SubClassName=ps_output  LeftPortType=input  RightPortType=output  PseudoPeriodic=off  Frequencies=[]  VectorFormat=1-D array  Unit=inherit  AffineConversion=off
      settings: SourceProductBaseCode=SS,PW,VE
  Spannungs-Mux : Mux  Inputs=10
  Strom-Mux : Mux  Inputs=10
  U{1..10} (10 alike) : fl_lib/Electrical/Electrical Sensors/Voltage Sensor
      settings: SourceProductBaseCode=PW,SS,VE
  L_in : PMIOPort  Side=Left
  N_in : PMIOPort  Port=2  Side=Left
  L_out : PMIOPort  Port=3  Side=Right
  N_out : PMIOPort  Port=4  Side=Right
  I_out : Outport
  U_out : Outport  Port=2
  wires:
  PS-Simulink Converter5/1 -> Strom-Mux/1  "I1"
  PS-Simulink Converter2/1 -> Strom-Mux/2  "I2"
  PS-Simulink Converter4/1 -> Strom-Mux/3  "I3"
  PS-Simulink Converter7/1 -> Strom-Mux/4  "I4"
  PS-Simulink Converter9/1 -> Strom-Mux/5  "I5"
  PS-Simulink Converter13/1 -> Strom-Mux/6  "I6"
  PS-Simulink Converter11/1 -> Strom-Mux/7  "I7"
  PS-Simulink Converter16/1 -> Strom-Mux/8  "I8"
  PS-Simulink Converter18/1 -> Strom-Mux/9  "I9"
  PS-Simulink Converter20/1 -> Strom-Mux/10  "I10"
  PS-Simulink Converter19/1 -> Spannungs-Mux/10  "U10"
  PS-Simulink Converter17/1 -> Spannungs-Mux/9  "U9"
  PS-Simulink Converter15/1 -> Spannungs-Mux/8  "U8"
  PS-Simulink Converter10/1 -> Spannungs-Mux/7  "U7"
  PS-Simulink Converter12/1 -> Spannungs-Mux/6  "U6"
  PS-Simulink Converter8/1 -> Spannungs-Mux/5  "U5"
  PS-Simulink Converter6/1 -> Spannungs-Mux/4  "U4"
  PS-Simulink Converter3/1 -> Spannungs-Mux/3  "U3"
  PS-Simulink Converter1/1 -> Spannungs-Mux/2  "U2"
  PS-Simulink Converter14/1 -> Spannungs-Mux/1  "U1"
  Strom-Mux/1 -> I_out/1
  Spannungs-Mux/1 -> U_out/1
  connections:
  U1/LConn1 -- L_in/RConn1 -- I1/LConn1
  N_in/RConn1 -- Leitungs-ESB 1/LConn2 -- U1/RConn2
  Leitungs-ESB 1/LConn1 -- I1/RConn2
  I1/RConn1 -- PS-Simulink Converter5/LConn1
  U1/RConn1 -- PS-Simulink Converter14/LConn1
  Leitungs-ESB 2/LConn2 -- U2/RConn2 -- Leitungs-ESB 1/RConn2
  U2/LConn1 -- I2/LConn1 -- Leitungs-ESB 1/RConn1
  I2/RConn1 -- PS-Simulink Converter2/LConn1
  U2/RConn1 -- PS-Simulink Converter1/LConn1
  U3/RConn2 -- Leitungs-ESB 3/LConn2 -- Leitungs-ESB 2/RConn2
  U3/LConn1 -- I3/LConn1 -- Leitungs-ESB 2/RConn1
  I3/RConn1 -- PS-Simulink Converter4/LConn1
  U3/RConn1 -- PS-Simulink Converter3/LConn1
  Leitungs-ESB 3/LConn1 -- I3/RConn2
  U4/RConn2 -- Leitungs-ESB 3/RConn2 -- Leitungs-ESB 4/LConn2
  U4/LConn1 -- Leitungs-ESB 3/RConn1 -- I4/LConn1
  I4/RConn1 -- PS-Simulink Converter7/LConn1
  U4/RConn1 -- PS-Simulink Converter6/LConn1
  Leitungs-ESB 4/RConn2 -- Leitungs-ESB 5/LConn2 -- U5/RConn2
  Leitungs-ESB 4/RConn1 -- I5/LConn1 -- U5/LConn1
  I5/RConn1 -- PS-Simulink Converter9/LConn1
  U5/RConn1 -- PS-Simulink Converter8/LConn1
  Leitungs-ESB 6/RConn2 -- Leitungs-ESB 7/LConn2 -- U7/RConn2
  Leitungs-ESB 6/RConn1 -- I7/LConn1 -- U7/LConn1
  I7/RConn1 -- PS-Simulink Converter11/LConn1
  U7/RConn1 -- PS-Simulink Converter10/LConn1
  Leitungs-ESB 6/LConn2 -- Leitungs-ESB 5/RConn2 -- U6/RConn2
  Leitungs-ESB 5/RConn1 -- I6/LConn1 -- U6/LConn1
  U6/RConn1 -- PS-Simulink Converter12/LConn1
  I6/RConn1 -- PS-Simulink Converter13/LConn1
  I6/RConn2 -- Leitungs-ESB 6/LConn1
  Leitungs-ESB 8/LConn2 -- Leitungs-ESB 7/RConn2 -- U8/RConn2
  Leitungs-ESB 7/RConn1 -- I8/LConn1 -- U8/LConn1
  I8/RConn1 -- PS-Simulink Converter16/LConn1
  U8/RConn1 -- PS-Simulink Converter15/LConn1
  Leitungs-ESB 8/RConn2 -- Leitungs-ESB 9/LConn2 -- U9/RConn2
  Leitungs-ESB 8/RConn1 -- I9/LConn1 -- U9/LConn1
  I9/RConn1 -- PS-Simulink Converter18/LConn1
  U9/RConn1 -- PS-Simulink Converter17/LConn1
  U10/RConn2 -- Leitungs-ESB 9/RConn2 -- Leitungs-ESB 10/LConn2
  Leitungs-ESB 9/RConn1 -- I10/LConn1 -- U10/LConn1
  I10/RConn1 -- PS-Simulink Converter20/LConn1
  U10/RConn1 -- PS-Simulink Converter19/LConn1
  Leitungs-ESB 10/RConn1 -- L_out/RConn1
  Leitungs-ESB 10/RConn2 -- N_out/RConn1
  I2/RConn2 -- Leitungs-ESB 2/LConn1
  Leitungs-ESB 4/LConn1 -- I4/RConn2
  I5/RConn2 -- Leitungs-ESB 5/LConn1
  I7/RConn2 -- Leitungs-ESB 7/LConn1
  I8/RConn2 -- Leitungs-ESB 8/LConn1
  I9/RConn2 -- Leitungs-ESB 9/LConn1
  I10/RConn2 -- Leitungs-ESB 10/LConn1

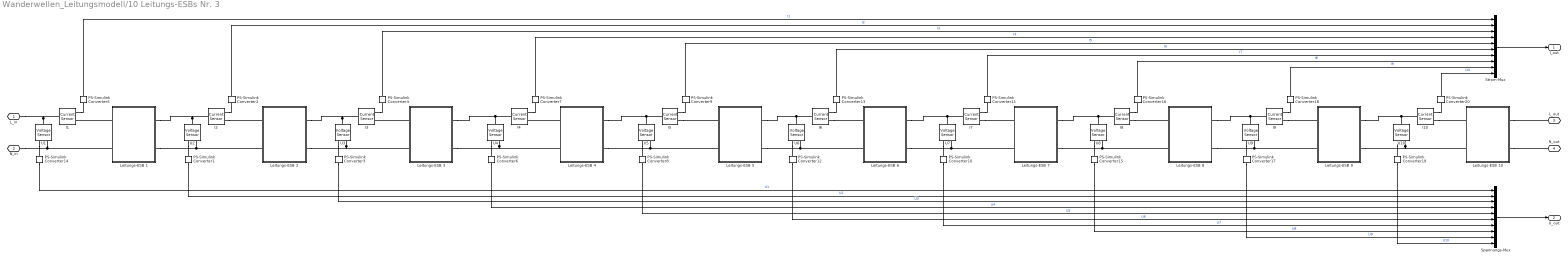
== system Wanderwellen_Leitungsmodell/10 Leitungs-ESBs Nr. 3 ==
  I{1..10} (10 alike) : fl_lib/Electrical/Electrical Sensors/Current Sensor
      settings: SourceProductBaseCode=PW,SS,VE
  Leitungs-ESB 1 : Subsystem
  Leitungs-ESB 10 : Subsystem
  Leitungs-ESB 2 : Subsystem
  Leitungs-ESB 3 : Subsystem
  Leitungs-ESB 4 : Subsystem
  Leitungs-ESB 5 : Subsystem
  Leitungs-ESB 6 : Subsystem
  Leitungs-ESB 7 : Subsystem
  Leitungs-ESB 8 : Subsystem
  Leitungs-ESB 9 : Subsystem
  PS-Simulink Converter{1..20} (20 alike) : nesl_utility/PS-Simulink Converter  PhysicalDomain=network_engine_domain  SubClassName=ps_output  LeftPortType=input  RightPortType=output  PseudoPeriodic=off  Frequencies=[]  VectorFormat=1-D array  Unit=inherit  AffineConversion=off
      settings: SourceProductBaseCode=SS,PW,VE
  Spannungs-Mux : Mux  Inputs=10
  Strom-Mux : Mux  Inputs=10
  U{1..10} (10 alike) : fl_lib/Electrical/Electrical Sensors/Voltage Sensor
      settings: SourceProductBaseCode=PW,SS,VE
  L_in : PMIOPort  Side=Left
  N_in : PMIOPort  Port=2  Side=Left
  L_out : PMIOPort  Port=3  Side=Right
  N_out : PMIOPort  Port=4  Side=Right
  I_out : Outport
  U_out : Outport  Port=2
  wires:
  PS-Simulink Converter5/1 -> Strom-Mux/1  "I1"
  PS-Simulink Converter2/1 -> Strom-Mux/2  "I2"
  PS-Simulink Converter4/1 -> Strom-Mux/3  "I3"
  PS-Simulink Converter7/1 -> Strom-Mux/4  "I4"
  PS-Simulink Converter9/1 -> Strom-Mux/5  "I5"
  PS-Simulink Converter13/1 -> Strom-Mux/6  "I6"
  PS-Simulink Converter11/1 -> Strom-Mux/7  "I7"
  PS-Simulink Converter16/1 -> Strom-Mux/8  "I8"
  PS-Simulink Converter18/1 -> Strom-Mux/9  "I9"
  PS-Simulink Converter20/1 -> Strom-Mux/10  "I10"
  PS-Simulink Converter19/1 -> Spannungs-Mux/10  "U10"
  PS-Simulink Converter17/1 -> Spannungs-Mux/9  "U9"
  PS-Simulink Converter15/1 -> Spannungs-Mux/8  "U8"
  PS-Simulink Converter10/1 -> Spannungs-Mux/7  "U7"
  PS-Simulink Converter12/1 -> Spannungs-Mux/6  "U6"
  PS-Simulink Converter8/1 -> Spannungs-Mux/5  "U5"
  PS-Simulink Converter6/1 -> Spannungs-Mux/4  "U4"
  PS-Simulink Converter3/1 -> Spannungs-Mux/3  "U3"
  PS-Simulink Converter1/1 -> Spannungs-Mux/2  "U2"
  PS-Simulink Converter14/1 -> Spannungs-Mux/1  "U1"
  Strom-Mux/1 -> I_out/1
  Spannungs-Mux/1 -> U_out/1
  connections:
  U1/LConn1 -- L_in/RConn1 -- I1/LConn1
  N_in/RConn1 -- Leitungs-ESB 1/LConn2 -- U1/RConn2
  Leitungs-ESB 1/LConn1 -- I1/RConn2
  I1/RConn1 -- PS-Simulink Converter5/LConn1
  U1/RConn1 -- PS-Simulink Converter14/LConn1
  Leitungs-ESB 2/LConn2 -- U2/RConn2 -- Leitungs-ESB 1/RConn2
  U2/LConn1 -- I2/LConn1 -- Leitungs-ESB 1/RConn1
  I2/RConn1 -- PS-Simulink Converter2/LConn1
  U2/RConn1 -- PS-Simulink Converter1/LConn1
  U3/RConn2 -- Leitungs-ESB 3/LConn2 -- Leitungs-ESB 2/RConn2
  U3/LConn1 -- I3/LConn1 -- Leitungs-ESB 2/RConn1
  I3/RConn1 -- PS-Simulink Converter4/LConn1
  U3/RConn1 -- PS-Simulink Converter3/LConn1
  Leitungs-ESB 3/LConn1 -- I3/RConn2
  U4/RConn2 -- Leitungs-ESB 3/RConn2 -- Leitungs-ESB 4/LConn2
  U4/LConn1 -- Leitungs-ESB 3/RConn1 -- I4/LConn1
  I4/RConn1 -- PS-Simulink Converter7/LConn1
  U4/RConn1 -- PS-Simulink Converter6/LConn1
  Leitungs-ESB 4/RConn2 -- Leitungs-ESB 5/LConn2 -- U5/RConn2
  Leitungs-ESB 4/RConn1 -- I5/LConn1 -- U5/LConn1
  I5/RConn1 -- PS-Simulink Converter9/LConn1
  U5/RConn1 -- PS-Simulink Converter8/LConn1
  Leitungs-ESB 6/RConn2 -- Leitungs-ESB 7/LConn2 -- U7/RConn2
  Leitungs-ESB 6/RConn1 -- I7/LConn1 -- U7/LConn1
  I7/RConn1 -- PS-Simulink Converter11/LConn1
  U7/RConn1 -- PS-Simulink Converter10/LConn1
  Leitungs-ESB 6/LConn2 -- Leitungs-ESB 5/RConn2 -- U6/RConn2
  Leitungs-ESB 5/RConn1 -- I6/LConn1 -- U6/LConn1
  U6/RConn1 -- PS-Simulink Converter12/LConn1
  I6/RConn1 -- PS-Simulink Converter13/LConn1
  I6/RConn2 -- Leitungs-ESB 6/LConn1
  Leitungs-ESB 8/LConn2 -- Leitungs-ESB 7/RConn2 -- U8/RConn2
  Leitungs-ESB 7/RConn1 -- I8/LConn1 -- U8/LConn1
  I8/RConn1 -- PS-Simulink Converter16/LConn1
  U8/RConn1 -- PS-Simulink Converter15/LConn1
  Leitungs-ESB 8/RConn2 -- Leitungs-ESB 9/LConn2 -- U9/RConn2
  Leitungs-ESB 8/RConn1 -- I9/LConn1 -- U9/LConn1
  I9/RConn1 -- PS-Simulink Converter18/LConn1
  U9/RConn1 -- PS-Simulink Converter17/LConn1
  U10/RConn2 -- Leitungs-ESB 9/RConn2 -- Leitungs-ESB 10/LConn2
  Leitungs-ESB 9/RConn1 -- I10/LConn1 -- U10/LConn1
  I10/RConn1 -- PS-Simulink Converter20/LConn1
  U10/RConn1 -- PS-Simulink Converter19/LConn1
  Leitungs-ESB 10/RConn1 -- L_out/RConn1
  Leitungs-ESB 10/RConn2 -- N_out/RConn1
  I2/RConn2 -- Leitungs-ESB 2/LConn1
  Leitungs-ESB 4/LConn1 -- I4/RConn2
  I5/RConn2 -- Leitungs-ESB 5/LConn1
  I7/RConn2 -- Leitungs-ESB 7/LConn1
  I8/RConn2 -- Leitungs-ESB 8/LConn1
  I9/RConn2 -- Leitungs-ESB 9/LConn1
  I10/RConn2 -- Leitungs-ESB 10/LConn1

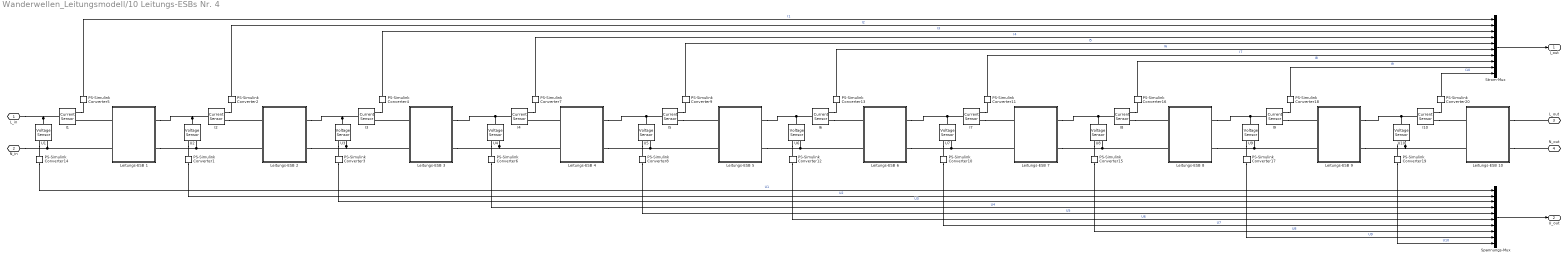
== system Wanderwellen_Leitungsmodell/10 Leitungs-ESBs Nr. 4 ==
  I{1..10} (10 alike) : fl_lib/Electrical/Electrical Sensors/Current Sensor
      settings: SourceProductBaseCode=PW,SS,VE
  Leitungs-ESB 1 : Subsystem
  Leitungs-ESB 10 : Subsystem
  Leitungs-ESB 2 : Subsystem
  Leitungs-ESB 3 : Subsystem
  Leitungs-ESB 4 : Subsystem
  Leitungs-ESB 5 : Subsystem
  Leitungs-ESB 6 : Subsystem
  Leitungs-ESB 7 : Subsystem
  Leitungs-ESB 8 : Subsystem
  Leitungs-ESB 9 : Subsystem
  PS-Simulink Converter{1..20} (20 alike) : nesl_utility/PS-Simulink Converter  PhysicalDomain=network_engine_domain  SubClassName=ps_output  LeftPortType=input  RightPortType=output  PseudoPeriodic=off  Frequencies=[]  VectorFormat=1-D array  Unit=inherit  AffineConversion=off
      settings: SourceProductBaseCode=SS,PW,VE
  Spannungs-Mux : Mux  Inputs=10
  Strom-Mux : Mux  Inputs=10
  U{1..10} (10 alike) : fl_lib/Electrical/Electrical Sensors/Voltage Sensor
      settings: SourceProductBaseCode=PW,SS,VE
  L_in : PMIOPort  Side=Left
  N_in : PMIOPort  Port=2  Side=Left
  L_out : PMIOPort  Port=3  Side=Right
  N_out : PMIOPort  Port=4  Side=Right
  I_out : Outport
  U_out : Outport  Port=2
  wires:
  PS-Simulink Converter5/1 -> Strom-Mux/1  "I1"
  PS-Simulink Converter2/1 -> Strom-Mux/2  "I2"
  PS-Simulink Converter4/1 -> Strom-Mux/3  "I3"
  PS-Simulink Converter7/1 -> Strom-Mux/4  "I4"
  PS-Simulink Converter9/1 -> Strom-Mux/5  "I5"
  PS-Simulink Converter13/1 -> Strom-Mux/6  "I6"
  PS-Simulink Converter11/1 -> Strom-Mux/7  "I7"
  PS-Simulink Converter16/1 -> Strom-Mux/8  "I8"
  PS-Simulink Converter18/1 -> Strom-Mux/9  "I9"
  PS-Simulink Converter20/1 -> Strom-Mux/10  "I10"
  PS-Simulink Converter19/1 -> Spannungs-Mux/10  "U10"
  PS-Simulink Converter17/1 -> Spannungs-Mux/9  "U9"
  PS-Simulink Converter15/1 -> Spannungs-Mux/8  "U8"
  PS-Simulink Converter10/1 -> Spannungs-Mux/7  "U7"
  PS-Simulink Converter12/1 -> Spannungs-Mux/6  "U6"
  PS-Simulink Converter8/1 -> Spannungs-Mux/5  "U5"
  PS-Simulink Converter6/1 -> Spannungs-Mux/4  "U4"
  PS-Simulink Converter3/1 -> Spannungs-Mux/3  "U3"
  PS-Simulink Converter1/1 -> Spannungs-Mux/2  "U2"
  PS-Simulink Converter14/1 -> Spannungs-Mux/1  "U1"
  Strom-Mux/1 -> I_out/1
  Spannungs-Mux/1 -> U_out/1
  connections:
  U1/LConn1 -- L_in/RConn1 -- I1/LConn1
  N_in/RConn1 -- Leitungs-ESB 1/LConn2 -- U1/RConn2
  Leitungs-ESB 1/LConn1 -- I1/RConn2
  I1/RConn1 -- PS-Simulink Converter5/LConn1
  U1/RConn1 -- PS-Simulink Converter14/LConn1
  Leitungs-ESB 2/LConn2 -- U2/RConn2 -- Leitungs-ESB 1/RConn2
  U2/LConn1 -- I2/LConn1 -- Leitungs-ESB 1/RConn1
  I2/RConn1 -- PS-Simulink Converter2/LConn1
  U2/RConn1 -- PS-Simulink Converter1/LConn1
  U3/RConn2 -- Leitungs-ESB 3/LConn2 -- Leitungs-ESB 2/RConn2
  U3/LConn1 -- I3/LConn1 -- Leitungs-ESB 2/RConn1
  I3/RConn1 -- PS-Simulink Converter4/LConn1
  U3/RConn1 -- PS-Simulink Converter3/LConn1
  Leitungs-ESB 3/LConn1 -- I3/RConn2
  U4/RConn2 -- Leitungs-ESB 3/RConn2 -- Leitungs-ESB 4/LConn2
  U4/LConn1 -- Leitungs-ESB 3/RConn1 -- I4/LConn1
  I4/RConn1 -- PS-Simulink Converter7/LConn1
  U4/RConn1 -- PS-Simulink Converter6/LConn1
  Leitungs-ESB 4/RConn2 -- Leitungs-ESB 5/LConn2 -- U5/RConn2
  Leitungs-ESB 4/RConn1 -- I5/LConn1 -- U5/LConn1
  I5/RConn1 -- PS-Simulink Converter9/LConn1
  U5/RConn1 -- PS-Simulink Converter8/LConn1
  Leitungs-ESB 6/RConn2 -- Leitungs-ESB 7/LConn2 -- U7/RConn2
  Leitungs-ESB 6/RConn1 -- I7/LConn1 -- U7/LConn1
  I7/RConn1 -- PS-Simulink Converter11/LConn1
  U7/RConn1 -- PS-Simulink Converter10/LConn1
  Leitungs-ESB 6/LConn2 -- Leitungs-ESB 5/RConn2 -- U6/RConn2
  Leitungs-ESB 5/RConn1 -- I6/LConn1 -- U6/LConn1
  U6/RConn1 -- PS-Simulink Converter12/LConn1
  I6/RConn1 -- PS-Simulink Converter13/LConn1
  I6/RConn2 -- Leitungs-ESB 6/LConn1
  Leitungs-ESB 8/LConn2 -- Leitungs-ESB 7/RConn2 -- U8/RConn2
  Leitungs-ESB 7/RConn1 -- I8/LConn1 -- U8/LConn1
  I8/RConn1 -- PS-Simulink Converter16/LConn1
  U8/RConn1 -- PS-Simulink Converter15/LConn1
  Leitungs-ESB 8/RConn2 -- Leitungs-ESB 9/LConn2 -- U9/RConn2
  Leitungs-ESB 8/RConn1 -- I9/LConn1 -- U9/LConn1
  I9/RConn1 -- PS-Simulink Converter18/LConn1
  U9/RConn1 -- PS-Simulink Converter17/LConn1
  U10/RConn2 -- Leitungs-ESB 9/RConn2 -- Leitungs-ESB 10/LConn2
  Leitungs-ESB 9/RConn1 -- I10/LConn1 -- U10/LConn1
  I10/RConn1 -- PS-Simulink Converter20/LConn1
  U10/RConn1 -- PS-Simulink Converter19/LConn1
  Leitungs-ESB 10/RConn1 -- L_out/RConn1
  Leitungs-ESB 10/RConn2 -- N_out/RConn1
  I2/RConn2 -- Leitungs-ESB 2/LConn1
  Leitungs-ESB 4/LConn1 -- I4/RConn2
  I5/RConn2 -- Leitungs-ESB 5/LConn1
  I7/RConn2 -- Leitungs-ESB 7/LConn1
  I8/RConn2 -- Leitungs-ESB 8/LConn1
  I9/RConn2 -- Leitungs-ESB 9/LConn1
  I10/RConn2 -- Leitungs-ESB 10/LConn1
